simulink model "a43_balance_model_verification"  (R2026a)
settings: Solver=ode45  StopTime=8
settings Model: Creator=ianhe  LastModifiedBy=ianhe

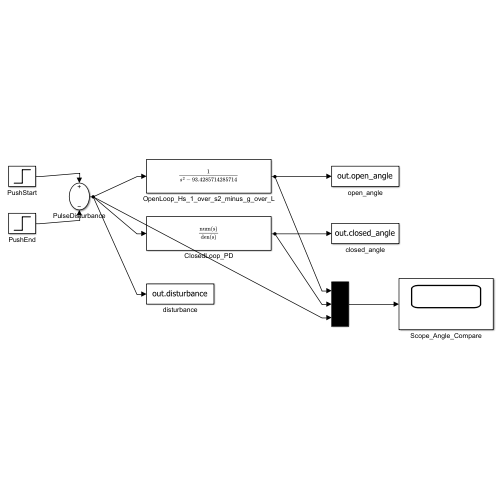
[thumbnail: Simulink's stored preview of the top-level diagram]
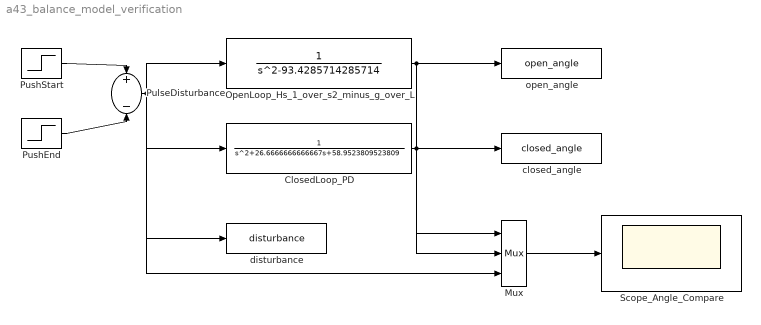
== system a43_balance_model_verification ==
  ClosedLoop_PD : TransferFcn  Denominator=[1 26.6666666666667 58.9523809523809]
  Mux : Mux  Inputs=3
  OpenLoop_Hs_1_over_s2_minus_g_over_L : TransferFcn  Denominator=[1 0 -93.4285714285714]
  PulseDisturbance : Sum  Inputs=+-
  PushEnd : Step  Time=4  SampleTime=0
  PushStart : Step  Time=3  SampleTime=0
  Scope_Angle_Compare : Scope
  closed_angle : ToWorkspace  VariableName=closed_angle  SaveFormat=Structure With Time  SampleTime=-1
  disturbance : ToWorkspace  VariableName=disturbance  SaveFormat=Structure With Time  SampleTime=-1
  open_angle : ToWorkspace  VariableName=open_angle  SaveFormat=Structure With Time  SampleTime=-1
  wires:
  PushStart/1 -> PulseDisturbance/1
  PushEnd/1 -> PulseDisturbance/2
  PulseDisturbance/1 -> OpenLoop_Hs_1_over_s2_minus_g_over_L/1, ClosedLoop_PD/1, disturbance/1, Mux/3
  OpenLoop_Hs_1_over_s2_minus_g_over_L/1 -> open_angle/1, Mux/1
  ClosedLoop_PD/1 -> closed_angle/1, Mux/2
  Mux/1 -> Scope_Angle_Compare/1
